simulink model "PenduloCausalidade"  (Simulink 7.5)
settings: Solver=ode45  StartTime=0.0  StopTime=100  RelTol=1e-3
settings Model: Creator=Leonardo  LastModifiedBy=Leo

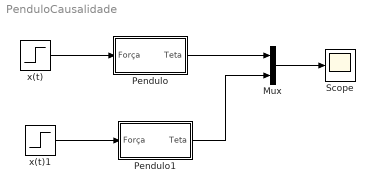
== system PenduloCausalidade ==
  Mux : Mux  Inputs=2
  Pendulo : Subsystem
  Pendulo1 : Subsystem
  Scope : Scope
      settings: TimeRange=100  YMin=0  YMax=1
  x(t) : Step  Time=50  Before=-1  SampleTime=0
  x(t)1 : Step  Time=50  Before=-1  After=-0.5  SampleTime=0
  wires:
  x(t)/1 -> Pendulo/1(Força)
  Mux/1 -> Scope/1
  Pendulo/1(Teta) -> Mux/1
  Pendulo1/1(Teta) -> Mux/2
  x(t)1/1 -> Pendulo1/1(Força)

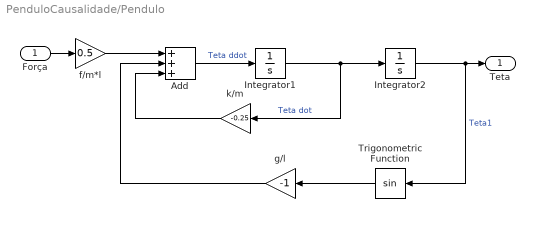
== system PenduloCausalidade/Pendulo ==
  Força : Inport
  Add : Sum  Inputs=+++
  Integrator1 : Integrator
  Integrator2 : Integrator
  Trigonometric Function : Trigonometry
  f/m*l : Gain  Gain=0.5
  g/l : Gain  Gain=-1
  k/m : Gain  Gain=-0.25
  Teta : Outport
  wires:
  Integrator1/1 -> Integrator2/1, k/m/1  "Teta dot"
  Add/1 -> Integrator1/1  "Teta ddot"
  Integrator2/1 -> Teta/1, Trigonometric Function/1  "Teta1"
  Trigonometric Function/1 -> g/l/1
  g/l/1 -> Add/2
  k/m/1 -> Add/3
  f/m*l/1 -> Add/1
  Força/1 -> f/m*l/1

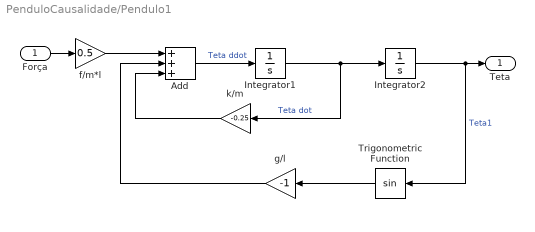
== system PenduloCausalidade/Pendulo1 ==
  Força : Inport
  Add : Sum  Inputs=+++
  Integrator1 : Integrator
  Integrator2 : Integrator
  Trigonometric Function : Trigonometry
  f/m*l : Gain  Gain=0.5
  g/l : Gain  Gain=-1
  k/m : Gain  Gain=-0.25
  Teta : Outport
  wires:
  Integrator1/1 -> Integrator2/1, k/m/1  "Teta dot"
  Add/1 -> Integrator1/1  "Teta ddot"
  Integrator2/1 -> Teta/1, Trigonometric Function/1  "Teta1"
  Trigonometric Function/1 -> g/l/1
  g/l/1 -> Add/2
  k/m/1 -> Add/3
  f/m*l/1 -> Add/1
  Força/1 -> f/m*l/1
